simulink model "Problem6"  (R2020b)
settings: Solver=VariableStepAuto  StartTime=0.0  StopTime=10.0  RelTol=1e-3
settings Model: Creator=Shirish  LastModifiedBy=Shirish

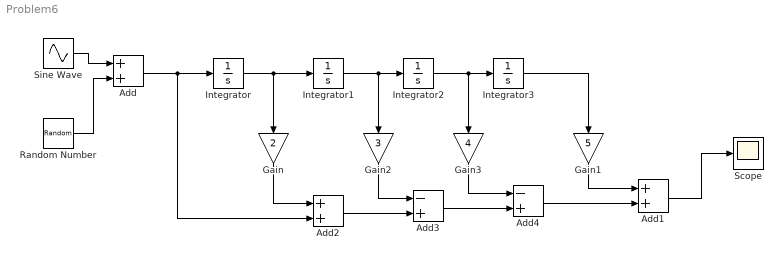
== system Problem6 ==
  Add : Sum
  Add1 : Sum
  Add2 : Sum
  Add3 : Sum  Inputs=-+
  Add4 : Sum  Inputs=-+
  Gain : Gain  Gain=2
  Gain1 : Gain  Gain=5
  Gain2 : Gain  Gain=3
  Gain3 : Gain  Gain=4
  Integrator{,1..3} (4 alike) : Integrator
  Random Number : RandomNumber  Variance=0.05  SampleTime=0.1
  Scope : Scope
  Sine Wave : Sin  SampleTime=0
  wires:
  Sine Wave/1 -> Add/1
  Random Number/1 -> Add/2
  Integrator/1 -> Gain/1, Integrator1/1
  Integrator1/1 -> Gain2/1, Integrator2/1
  Integrator2/1 -> Gain3/1, Integrator3/1
  Integrator3/1 -> Gain1/1
  Add2/1 -> Add3/2
  Gain2/1 -> Add3/1
  Gain/1 -> Add2/1
  Add/1 -> Add2/2, Integrator/1
  Gain3/1 -> Add4/1
  Add3/1 -> Add4/2
  Gain1/1 -> Add1/1
  Add4/1 -> Add1/2
  Add1/1 -> Scope/1
